simulink model "L3_1_P_control"  (R2025b)
settings: Solver=VariableStepAuto  StartTime=0.0  StopTime=5  RelTol=1e-3
settings Model: Creator=kimsteph  LastModifiedBy=kimsteph

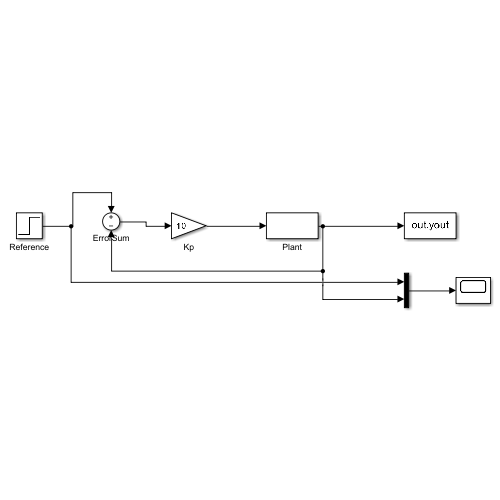
[thumbnail: Simulink's stored preview of the top-level diagram]
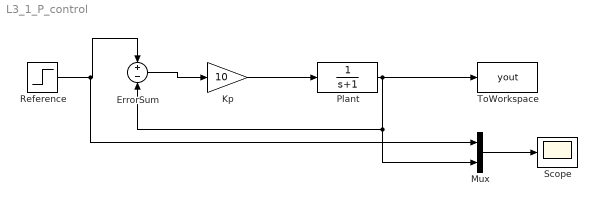
== system L3_1_P_control ==
  ErrorSum : Sum  Inputs=+-
  Kp : Gain  Gain=10
  Mux : Mux  Inputs=2
  Plant : TransferFcn  Denominator=[1 1]
  Reference : Step  SampleTime=0
  Scope : Scope
  ToWorkspace : ToWorkspace  VariableName=yout  SaveFormat=Timeseries  SampleTime=-1
  wires:
  Reference/1 -> ErrorSum/1, Mux/1
  ErrorSum/1 -> Kp/1
  Kp/1 -> Plant/1
  Plant/1 -> ErrorSum/2, Mux/2, ToWorkspace/1
  Mux/1 -> Scope/1
